simulink model "SIMULINK_EX_I"  (R2021a)
settings: Solver=VariableStepAuto  StartTime=0.0  StopTime=10.0  RelTol=1e-3
settings Model: Creator=GHOST  LastModifiedBy=GHOST

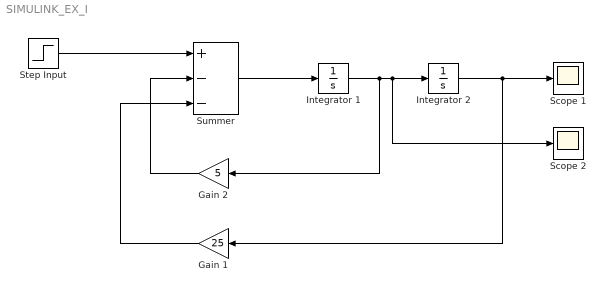
== system SIMULINK_EX_I ==
  Gain 1 : Gain  Gain=25
  Gain 2 : Gain  Gain=5
  Integrator 1 : Integrator
  Integrator 2 : Integrator
  Scope 1 : Scope
  Scope 2 : Scope
  Step Input : Step  Time=100  Before=25  After=25  SampleTime=0
  Summer : Sum  Inputs=+--
  wires:
  Step Input/1 -> Summer/1
  Gain 2/1 -> Summer/2
  Gain 1/1 -> Summer/3
  Summer/1 -> Integrator 1/1
  Integrator 1/1 -> Gain 2/1, Integrator 2/1, Scope 2/1
  Integrator 2/1 -> Gain 1/1, Scope 1/1
